simulink model "model1"  (R2018a)
settings: Solver=VariableStepAuto  StartTime=0.0  StopTime=160  RelTol=1e-3
settings Model: Creator=Thoriqul Aziz  LastModifiedBy=Thoriqul Aziz

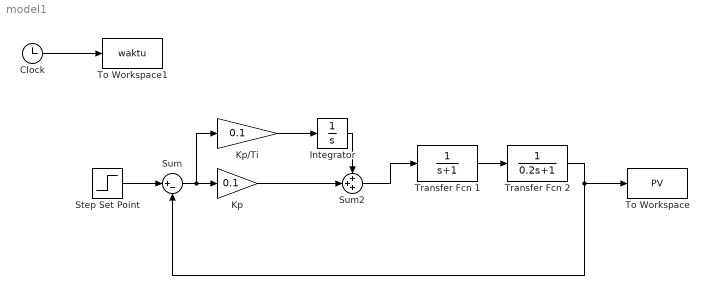
== system model1 ==
  Clock : Clock
  Integrator : Integrator
  Kp : Gain  Gain=0.1
  Kp/Ti : Gain  Gain=0.1
  Step Set Point : Step  SampleTime=0.1
  Sum : Sum  Inputs=|+-
  Sum2 : Sum  Inputs=+++
  To Workspace : ToWorkspace  VariableName=PV  SampleTime=-1
  To Workspace1 : ToWorkspace  VariableName=waktu  SampleTime=0.1
  Transfer Fcn 1 : TransferFcn  Denominator=[1 1]
  Transfer Fcn 2 : TransferFcn  Denominator=[0.2 1]
  wires:
  Step Set Point/1 -> Sum/1
  Sum/1 -> Kp/Ti/1, Kp/1
  Kp/Ti/1 -> Integrator/1
  Kp/1 -> Sum2/2
  Integrator/1 -> Sum2/1
  Sum2/1 -> Transfer Fcn 1/1
  Clock/1 -> To Workspace1/1
  Transfer Fcn 1/1 -> Transfer Fcn 2/1
  Transfer Fcn 2/1 -> To Workspace/1, Sum/2
